simulink model "gm_lab2_01"  (R2022a)
settings: Solver=VariableStepAuto  StartTime=0.0  StopTime=10.0  RelTol=1e-3
settings Model: Creator=Illia  LastModifiedBy=Illia
settings OptimizationCC: BlockReduction=off  ConditionallyExecuteInputs=off
settings DebuggingCC: InheritedTsInSrcMsg=none

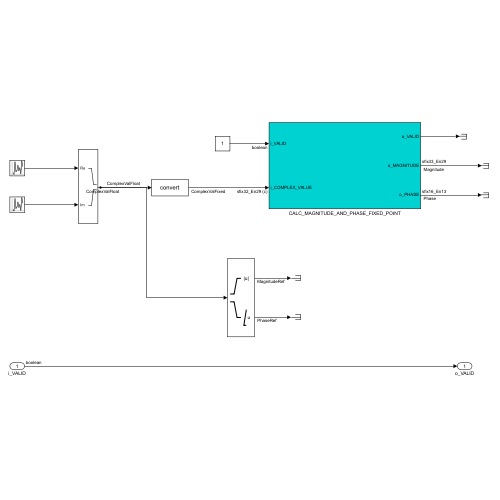
[thumbnail: Simulink's stored preview of the top-level diagram]
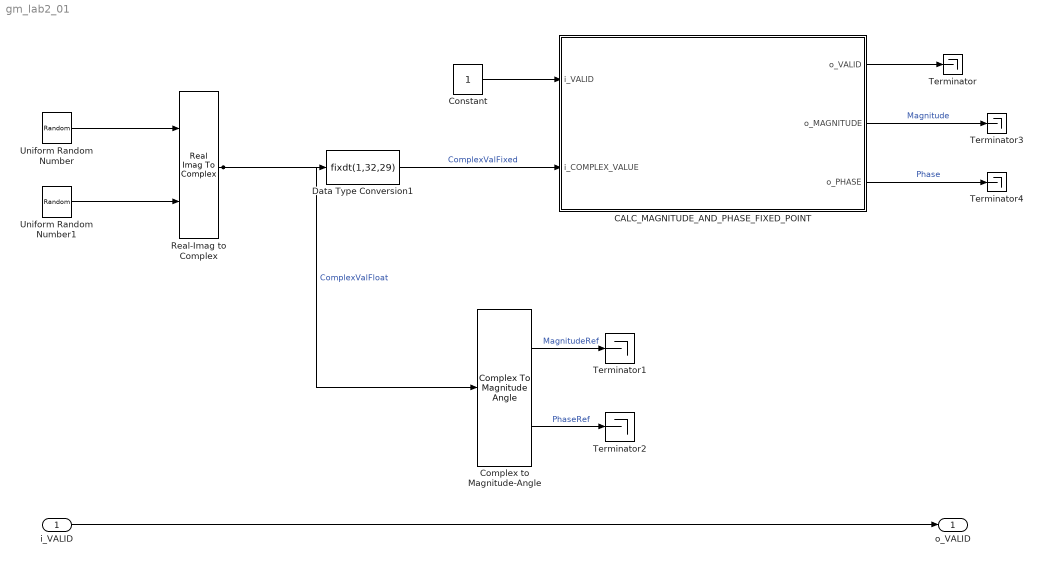
== system gm_lab2_01 ==
  i_VALID : Inport  OutDataTypeStr=boolean
  CALC_MAGNITUDE_AND_PHASE_FIXED_POINT : Subsystem
  Complex to Magnitude-Angle : ComplexToMagnitudeAngle
  Constant : Constant  OutDataTypeStr=boolean  SampleTime=1
  Data Type Conversion1 : DataTypeConversion  OutDataTypeStr=fixdt(1,32,29)  RndMeth=Round  SaturateOnIntegerOverflow=off
  Real-Imag to Complex : RealImagToComplex
  Terminator{,1..4} (5 alike) : Terminator
  Uniform Random Number : UniformRandomNumber  Minimum=-4  Maximum=4  Seed=3  SampleTime=1
  Uniform Random Number1 : UniformRandomNumber  Minimum=-4  Maximum=4  Seed=4  SampleTime=1
  o_VALID : Outport  VectorParamsAs1DForOutWhenUnconnected=off
  wires:
  i_VALID/1 -> o_VALID/1
  CALC_MAGNITUDE_AND_PHASE_FIXED_POINT/2(o_MAGNITUDE) -> Terminator3/1  "Magnitude"
  CALC_MAGNITUDE_AND_PHASE_FIXED_POINT/3(o_PHASE) -> Terminator4/1  "Phase"
  CALC_MAGNITUDE_AND_PHASE_FIXED_POINT/1(o_VALID) -> Terminator/1
  Constant/1 -> CALC_MAGNITUDE_AND_PHASE_FIXED_POINT/1(i_VALID)
  Data Type Conversion1/1 -> CALC_MAGNITUDE_AND_PHASE_FIXED_POINT/2(i_COMPLEX_VALUE)  "ComplexValFixed"
  Complex to Magnitude-Angle/2 -> Terminator2/1  "PhaseRef"
  Complex to Magnitude-Angle/1 -> Terminator1/1  "MagnitudeRef"
  Real-Imag to Complex/1 -> Complex to Magnitude-Angle/1, Data Type Conversion1/1  "ComplexValFloat"
  Uniform Random Number/1 -> Real-Imag to Complex/1
  Uniform Random Number1/1 -> Real-Imag to Complex/2

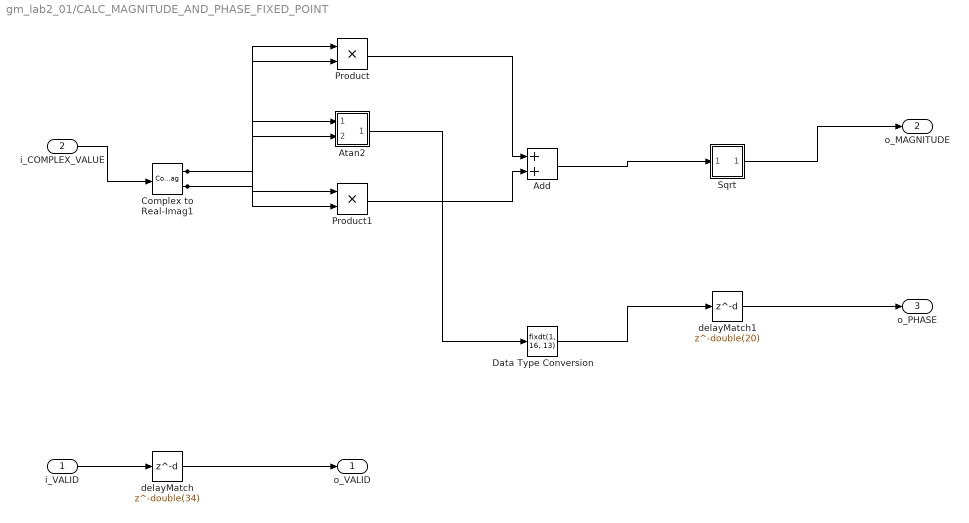
== system gm_lab2_01/CALC_MAGNITUDE_AND_PHASE_FIXED_POINT ==
  i_VALID : Inport  OutDataTypeStr=boolean  PortDimensions=1  SampleTime=1
  i_COMPLEX_VALUE : Inport  Port=2  OutDataTypeStr=fixdt(1, 32, 29)  PortDimensions=1  SampleTime=1
      settings: SignalType=complex
  Add : Sum  AccumDataTypeStr=fixdt(1, 64, 58)  OutDataTypeStr=fixdt(1, 64, 58)  SampleTime=1
  Atan2 : Subsystem
  Complex to Real-Imag1 : ComplexToRealImag  SampleTime=1
  Data Type Conversion : DataTypeConversion  OutDataTypeStr=fixdt(1, 16, 13)  RndMeth=Round  SampleTime=1  SaturateOnIntegerOverflow=off
  Product : Product  Inputs=**  OutDataTypeStr=fixdt(1, 64, 58)  SampleTime=1
  Product1 : Product  Inputs=**  OutDataTypeStr=fixdt(1, 64, 58)  SampleTime=1
  Sqrt : Subsystem
  delayMatch : Delay  DelayLength=double(34)  InitialCondition=0  SampleTime=1
  delayMatch1 : Delay  DelayLength=double(20)  InitialCondition=0  SampleTime=1
  o_VALID : Outport  SampleTime=1  VectorParamsAs1DForOutWhenUnconnected=off
  o_MAGNITUDE : Outport  Port=2  OutDataTypeStr=fixdt(1,33,29)  SampleTime=1
  o_PHASE : Outport  Port=3  OutDataTypeStr=fixdt(1,16,13)  SampleTime=1
  wires:
  delayMatch/1 -> o_VALID/1
  i_COMPLEX_VALUE/1 -> Complex to Real-Imag1/1
  Add/1 -> Sqrt/1(In1)
  Atan2/1(Out1) -> Data Type Conversion/1
  Complex to Real-Imag1/1 -> Product/2, Product/1, Atan2/2(In2)
  Complex to Real-Imag1/2 -> Product1/2, Product1/1, Atan2/1(In1)
  delayMatch1/1 -> o_PHASE/1
  Product/1 -> Add/1
  Product1/1 -> Add/2
  Sqrt/1(Out1) -> o_MAGNITUDE/1
  i_VALID/1 -> delayMatch/1
  Data Type Conversion/1 -> delayMatch1/1

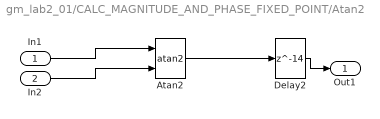
== system gm_lab2_01/CALC_MAGNITUDE_AND_PHASE_FIXED_POINT/Atan2 ==
  In1 : Inport
  In2 : Inport  Port=2
  Atan2 : Trigonometry  Operator=atan2  ApproximationMethod=CORDIC
  Delay2 : Delay  DelayLength=14
  Out1 : Outport
  wires:
  In1/1 -> Atan2/1
  In2/1 -> Atan2/2
  Atan2/1 -> Delay2/1
  Delay2/1 -> Out1/1

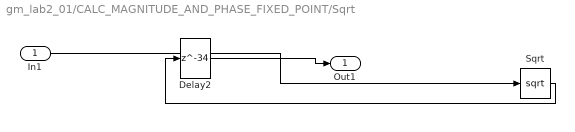
== system gm_lab2_01/CALC_MAGNITUDE_AND_PHASE_FIXED_POINT/Sqrt ==
  In1 : Inport
  Delay2 : Delay  DelayLength=34
  Sqrt : Sqrt  OutDataTypeStr=fixdt(1,33,29)
  Out1 : Outport
  wires:
  In1/1 -> Sqrt/1
  Sqrt/1 -> Delay2/1
  Delay2/1 -> Out1/1
